simulink model "DC_7a"  (R2022b)
settings: Solver=VariableStepAuto  StartTime=0.0  StopTime=tsim  RelTol=1e-3
undefined symbols (not defined in the file or in its folder): ts
libraries: cstblocks x3, simulink x1
settings Model: Creator=alici  LastModifiedBy=alici

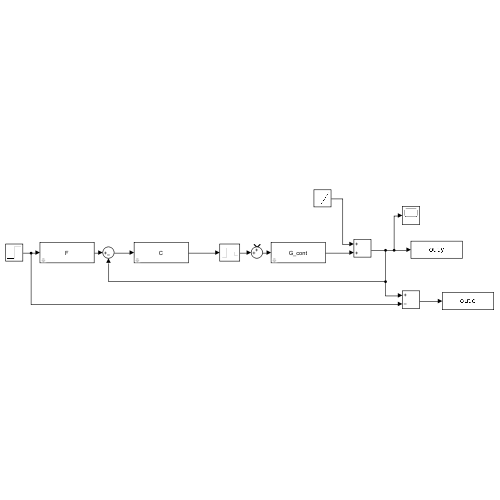
[thumbnail: Simulink's stored preview of the top-level diagram]
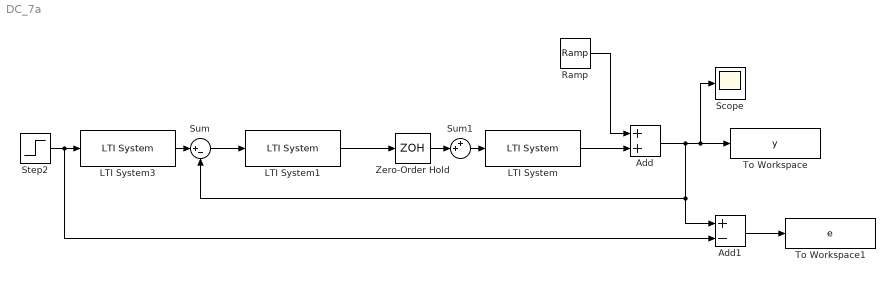
== system DC_7a ==
  Add : Sum
  Add1 : Sum  Inputs=+-
  LTI System : cstblocks/LTI System  sys=G_cont  IC=[]
  LTI System1 : cstblocks/LTI System  sys=C  IC=[]
  LTI System3 : cstblocks/LTI System  sys=F  IC=[]
  Ramp : simulink/Sources/Ramp  slope=0  start=0  InitialOutput=0
  Scope : Scope
  Step2 : Step  Time=0  SampleTime=0
  Sum : Sum  Inputs=|+-
  Sum1 : Sum  Inputs=++|
  To Workspace : ToWorkspace  VariableName=y  SaveFormat=Timeseries  SampleTime=ts/1000
  To Workspace1 : ToWorkspace  VariableName=e  SaveFormat=Timeseries  SampleTime=ts/1000
  Zero-Order Hold : ZeroOrderHold  SampleTime=ts
  wires:
  LTI System1/1 -> Zero-Order Hold/1
  Zero-Order Hold/1 -> Sum1/2
  Sum1/1 -> LTI System/1
  Sum/1 -> LTI System1/1
  LTI System/1 -> Add/2
  LTI System3/1 -> Sum/1
  Step2/1 -> Add1/2, LTI System3/1
  Ramp/1 -> Add/1
  Add/1 -> Sum/2, Add1/1, Scope/1, To Workspace/1
  Add1/1 -> To Workspace1/1
